simulink model "stepRecovery_compatibility"  (Simulink 8.3)
settings: Solver=ode3  SolverMode=SingleTasking  StartTime=0.0  StopTime="CONFIG.SIMULATION_TIME "  FixedStep=CONFIG.Ts  RelTol=1e-3
InitFcn:
  | cd(fileparts(which(bdroot)));
  | initStepRecovery;
values from neighbouring files (symbols this model uses):
  baseToWorldRotationPort = '/matlabTorqueBalancing/floatingBaseRotationMatrix:i'    [esperimento_fake2.mat]    (also in initStepRecovery.m = ['/' WBT_modelName '/floatingBaseRotationMatrix:i']; initTorqueBalancing.m = ['/' WBT_modelName '/floatingBaseRotationMatrix:i']; secondo_risultato.mat)
  bVectorConstraints = [0 0 0 0 0 0 0 0 0 0 0 0 ... (19 elements, 19x1)]    [esperimento_fake2.mat]    (also in secondo_risultato.mat)
  CONFIG =     [esperimento_fake2.mat]    (also in secondo_risultato.mat)
  ConstraintsMatrix = [3.73205080757 1 0.267949192431 -0.267949192431 -1 -3.73205080757 -3.73205080757 -1 -0.267949192431 0.267949192431 1 3.73205080757 ... (114 elements, 19x6)]    [esperimento_fake2.mat]    (also in secondo_risultato.mat)
  gain =     [esperimento_fake2.mat]    (also in secondo_risultato.mat)
  references =     [esperimento_fake2.mat]    (also in secondo_risultato.mat)
  reg =     [esperimento_fake2.mat]    (also in secondo_risultato.mat)
  ROBOT_DOF = 23    [esperimento_fake2.mat]    (also in secondo_risultato.mat)
  ROBOT_DOF_FOR_SIMULINK = [1 0 0 0 0 0 0 0 0 0 0 0 ... (529 elements, 23x23)]    [esperimento_fake2.mat]    (also in secondo_risultato.mat)
  sat =     [esperimento_fake2.mat]    (also in secondo_risultato.mat)
  SM =     [esperimento_fake2.mat]    (also in secondo_risultato.mat)
  sm =     [esperimento_fake2.mat]    (also in secondo_risultato.mat)
  WBT_modelName = 'matlabTorqueBalancing'    [esperimento_fake2.mat]    (also in initStepRecovery.m; initTorqueBalancing.m; secondo_risultato.mat)
  WBT_robotName = ''    [esperimento_fake2.mat]    (also in secondo_risultato.mat)
undefined symbols (not defined in the file or in its folder): bVectorConstraintsMPC, ConstraintsMatrixMPC, DiscIntNeverNeededParam, mpc_init
libraries: WBToolboxLibrary x191, simulink x22, simulink_extras x4
(part 6 of 6)

== system stepRecovery_compatibility/DesValues/State Machine Step Recovery/Step Recovery reference generator/Step Recovery Techniques /Capture Point Computer/Capture Point-alternative/omega ==
  COMx : Inport
  Constant : Constant  Value=9.81
  Divide : Product  Inputs=*/
  Selector : Selector  InputPortWidth=3  IndexOptions=Index vector (dialog)  Indices=[3]  OutputSizes=1
  Sqrt : Sqrt  SaturateOnIntegerOverflow=on
  holder 1 : WBToolboxLibrary/Utilities/holder 
  omega : Outport
  wires:
  Sqrt/1 -> omega/1
  Divide/1 -> Sqrt/1
  Constant/1 -> Divide/1
  holder 1/1 -> Divide/2
  Selector/1 -> holder 1/1
  COMx/1 -> Selector/1

== system stepRecovery_compatibility/DesValues/State Machine Step Recovery/Step Recovery reference generator/Step Recovery Techniques /Capture Point Computer/ICP /omega ==
  COMx : Inport
  Constant : Constant  Value=9.81
  Divide : Product  Inputs=*/
  Selector : Selector  InputPortWidth=3  IndexOptions=Index vector (dialog)  Indices=[3]  OutputSizes=1
  Sqrt : Sqrt  SaturateOnIntegerOverflow=on
  holder 1 : WBToolboxLibrary/Utilities/holder 
  omega : Outport
  wires:
  COMx/1 -> Selector/1
  Selector/1 -> holder 1/1
  holder 1/1 -> Divide/2
  Constant/1 -> Divide/1
  Divide/1 -> Sqrt/1
  Sqrt/1 -> omega/1

== system stepRecovery_compatibility/DesValues/State Machine Step Recovery/Step Recovery reference generator/Inverse Kinematics/Pseudo-Inverse kinematics Solver/From guess to q_ikin/l_sole_H_root_link1/Visualize hom transf4 ==
  H : Inport
  "CoM6D ->  CoMXYZ1" : Selector  NumberOfDimensions=2  InputPortWidth=7  IndexOptions=Index vector (dialog),Index vector (dialog)  Indices=[1 2 3],[1 2 3]  OutputSizes=1,1
  "CoM6D ->  CoMXYZ2" : Selector  NumberOfDimensions=2  InputPortWidth=7  IndexOptions=Index vector (dialog),Index vector (dialog)  Indices=[1 2 3],[4]  OutputSizes=1,1
  Hom : Scope
      settings: TimeRange=auto  ShowLegends=on  MaxDataPoints=5000  SaveToWorkspace=off  SaveName=ScopeData3  YMin=-1.25  YMax=1.25  SampleTime=-1
  R : Scope
      settings: TimeRange=auto  MaxDataPoints=5000  SaveToWorkspace=off  YMin=-0.125  YMax=1.125  SampleTime=-1
  p : Scope
      settings: TimeRange=auto  MaxDataPoints=5000  SaveToWorkspace=off  SaveName=ScopeData2  YMin=-1.00000  YMax=1.00000  SampleTime=-1
  wires:
  H/1 -> "CoM6D ->  CoMXYZ1"/1, Hom/1, "CoM6D ->  CoMXYZ2"/1
  "CoM6D ->  CoMXYZ2"/1 -> p/1
  "CoM6D ->  CoMXYZ1"/1 -> R/1

== system stepRecovery_compatibility/DesValues/State Machine Step Recovery/Step Recovery reference generator/Inverse Kinematics/Pseudo-Inverse kinematics Solver/From guess to q_ikin/l_sole_H_root_link2/Visualize hom transf4 ==
  H : Inport
  "CoM6D ->  CoMXYZ1" : Selector  NumberOfDimensions=2  InputPortWidth=7  IndexOptions=Index vector (dialog),Index vector (dialog)  Indices=[1 2 3],[1 2 3]  OutputSizes=1,1
  "CoM6D ->  CoMXYZ2" : Selector  NumberOfDimensions=2  InputPortWidth=7  IndexOptions=Index vector (dialog),Index vector (dialog)  Indices=[1 2 3],[4]  OutputSizes=1,1
  Hom : Scope
      settings: TimeRange=auto  ShowLegends=on  MaxDataPoints=5000  SaveToWorkspace=off  SaveName=ScopeData3  YMin=-1.25  YMax=1.25  SampleTime=-1
  R : Scope
      settings: TimeRange=auto  MaxDataPoints=5000  SaveToWorkspace=off  YMin=-0.125  YMax=1.125  SampleTime=-1
  p : Scope
      settings: TimeRange=auto  MaxDataPoints=5000  SaveToWorkspace=off  SaveName=ScopeData2  YMin=-1.00000  YMax=1.00000  SampleTime=-1
  wires:
  H/1 -> "CoM6D ->  CoMXYZ1"/1, Hom/1, "CoM6D ->  CoMXYZ2"/1
  "CoM6D ->  CoMXYZ2"/1 -> p/1
  "CoM6D ->  CoMXYZ1"/1 -> R/1

== matlab function DesValues/State Machine/visualise inertial/w_H_root_link1/fromImuToHomogeousTransformFCN ==
  data: imu_H_link input double; imu_H_link_0 input double; link_H_root input double; inertial_0 input double; inertial input double; neck input double; w_H_root output double; CONFIG parameter double
function w_H_root = fromBaseToWorldWithImuFCN(imu_H_link,imu_H_link_0,link_H_root,inertial_0,inertial,neck,CONFIG)
%#codegen
w_H_root = fromBaseToWorldWithImu(imu_H_link,imu_H_link_0,link_H_root,inertial_0,inertial,neck,CONFIG);

== matlab function DesValues/Internal coordinator/w_H_root_link4/fromImuToHomogeousTransformFCN ==
  data: imu_H_link input double; imu_H_link_0 input double; link_H_root input double; inertial_0 input double; inertial input double; neck input double; w_H_root output double; CONFIG parameter double
function w_H_root = fromBaseToWorldWithImuFCN(imu_H_link,imu_H_link_0,link_H_root,inertial_0,inertial,neck,CONFIG)
%#codegen
w_H_root = fromBaseToWorldWithImu(imu_H_link,imu_H_link_0,link_H_root,inertial_0,inertial,neck,CONFIG);

== matlab function DesValues/MATLAB Function ==
  data: w_H_b_vectorised input double; w_H_b output double; foot_p_b input double; rollPitchYaw output double
function [w_H_b,rollPitchYaw] = buildHomogenousTranformation(w_H_b_vectorised,foot_p_b)
%#codegen

w_H_b = [w_H_b_vectorised(1:4),w_H_b_vectorised(5:8),w_H_b_vectorised(9:12),...
         w_H_b_vectorised(13:16)];

w_H_b(1:3,4) = foot_p_b;
rollPitchYaw = rollPitchYawFromRotation(w_H_b(1:3,1:3));
rollPitchYaw(3) = 0;

== matlab function controller_QP/integralOf Hw/MATLAB Function ==
  data: qjErr input double; dqjEquivalent output double; Jc input double; vbEquivalent output double
function [dqjEquivalent, vbEquivalent] = generateReferencesForH(qjErr,Jc)
%#codegen

dqjEquivalent = qjErr;
vbEquivalent  = -eye(6)/Jc(1:6,1:6)*Jc(1:6,7:end)*qjErr;

end

== matlab function DesValues/State Machine Walking/nu/MATLAB Function ==
  data: JcLeftFoot input double; JcRightFoot input double; activeFeetConstraints input double; y output double; qD input double; reg parameter double
function y = fcn(JcLeftFoot,JcRightFoot,activeFeetConstraints,qD,reg)
%#codegen

Jc = [activeFeetConstraints(1)*JcLeftFoot;
      activeFeetConstraints(2)*JcRightFoot];

pinvJb = (Jc(:,1:6)'*Jc(:,1:6) + reg.pinvDampVb*eye(6))\Jc(:,1:6)';  
  
% pinvJb = pinv(Jc(:,1:6));

y = -pinvJb*Jc(:,7:end)*qD;

== matlab function DesValues/State Machine Walking/stateMachineFCN ==
  data: connection input double; wrench_rightFoot input double; wrench_leftFoot input double; CoM_0 input double; q0 input double; w_CoM input double; CoMIn input double; qIn input double; constraintsIn input double; w_H_b output double; CoMDes output double; qDes output double; constraints output double; l_sole_H_b input double; r_sole_H_b input double; sm parameter double; impedances output double; gain parameter double; currentState output double
function [w_H_b, CoMDes,qDes,constraints,impedances,currentState] = ...
    stateMachineFCN(connection,wrench_rightFoot,wrench_leftFoot,CoM_0, q0, w_CoM , CoMIn, qIn, constraintsIn, l_sole_H_b, r_sole_H_b, sm,gain)
%#codegen
 
[CoMDes,qDes,constraints, currentState,impedances,w_H_b] = ...
    stateMachineWalking(connection,CoM_0, q0, w_CoM, CoMIn, qIn, constraintsIn, wrench_rightFoot,wrench_leftFoot,l_sole_H_b, r_sole_H_b, sm,gain);

== matlab function DesValues/Internal coordinator/nu/MATLAB Function ==
  data: JcLeftFoot input double; JcRightFoot input double; activeFeetConstraints input double; y output double; qD input double; reg parameter double
function y = fcn(JcLeftFoot,JcRightFoot,activeFeetConstraints,qD,reg)
%#codegen

Jc = [activeFeetConstraints(1)*JcLeftFoot;
      activeFeetConstraints(2)*JcRightFoot];

pinvJb = (Jc(:,1:6)'*Jc(:,1:6) + reg.pinvDampVb*eye(6))\Jc(:,1:6)';  
  
% pinvJb = pinv(Jc(:,1:6));

y = -pinvJb*Jc(:,7:end)*qD;

== matlab function DesValues/State Machine/w_H_root_link4/fromImuToHomogeousTransformFCN ==
  data: imu_H_link input double; imu_H_link_0 input double; link_H_root input double; inertial_0 input double; inertial input double; neck input double; w_H_root output double; CONFIG parameter double
function w_H_root = fromBaseToWorldWithImuFCN(imu_H_link,imu_H_link_0,link_H_root,inertial_0,inertial,neck,CONFIG)
%#codegen
w_H_root = fromBaseToWorldWithImu(imu_H_link,imu_H_link_0,link_H_root,inertial_0,inertial,neck,CONFIG);

== matlab function DesValues/State Machine/w_H_root_link1/fromImuToHomogeousTransformFCN ==
  data: imu_H_link input double; imu_H_link_0 input double; link_H_root input double; inertial_0 input double; inertial input double; neck input double; w_H_root output double; CONFIG parameter double
function w_H_root = fromBaseToWorldWithImuFCN(imu_H_link,imu_H_link_0,link_H_root,inertial_0,inertial,neck,CONFIG)
%#codegen
w_H_root = fromBaseToWorldWithImu(imu_H_link,imu_H_link_0,link_H_root,inertial_0,inertial,neck,CONFIG);

== matlab function DesValues/Internal coordinator/refGen/refGenFCN ==
  data: xCom0 input double; qDes output double; q0 input double; t input double; references parameter double; desired_x_dx_ddx_CoM output double
function [qDes,desired_x_dx_ddx_CoM] = refGenFCN(xCom0,q0,t,references)
%#codegen

[qDes,desired_x_dx_ddx_CoM] = refGen(xCom0,q0,t,references);

== matlab function DesValues/State Machine Walking/w_H_root_link4/fromImuToHomogeousTransformFCN ==
  data: imu_H_link input double; imu_H_link_0 input double; link_H_root input double; inertial_0 input double; inertial input double; neck input double; w_H_root output double; CONFIG parameter double
function w_H_root = fromBaseToWorldWithImuFCN(imu_H_link,imu_H_link_0,link_H_root,inertial_0,inertial,neck,CONFIG)
%#codegen
w_H_root = fromBaseToWorldWithImu(imu_H_link,imu_H_link_0,link_H_root,inertial_0,inertial,neck,CONFIG);

== matlab function DesValues/State Machine/nu/MATLAB Function ==
  data: JcLeftFoot input double; JcRightFoot input double; activeFeetConstraints input double; y output double; qD input double; reg parameter double
function y = fcn(JcLeftFoot,JcRightFoot,activeFeetConstraints,qD,reg)
%#codegen

Jc = [activeFeetConstraints(1)*JcLeftFoot;
      activeFeetConstraints(2)*JcRightFoot];

pinvJb = pinvDamped(Jc(:,1:6),reg.pinvDampVb);  
  
% pinvJb = pinv(Jc(:,1:6));

y = -pinvJb*Jc(:,7:end)*qD;

== matlab function DesValues/State Machine/stateMachineFCN ==
  data: wrench_rightFoot input double; wrench_leftFoot input double; w_H_b output double; CoMDes output double; qDes output double; constraints output double; CoM_0 input double; q0 input double; l_sole_CoM input double; r_sole_CoM input double; qj input double; t input double; l_sole_H_b input double; r_sole_H_b input double; sm parameter double; impedances output double; kpCom output double; kdCom output double; gain parameter double; currentState output double; jointsSmoothingTime output double
function [w_H_b, CoMDes,qDes,constraints,impedances,kpCom,kdCom,currentState,jointsSmoothingTime] = ...
    stateMachineFCN(wrench_rightFoot,wrench_leftFoot,CoM_0, q0, l_sole_CoM,r_sole_CoM,qj, t, l_sole_H_b, r_sole_H_b, sm,gain)
%#codegen
 
[w_H_b, CoMDes,qDes,constraints,impedances,kpCom,kdCom,currentState,jointsSmoothingTime] = ...
    stateMachine(CoM_0, q0, l_sole_CoM,r_sole_CoM,qj, t, wrench_rightFoot,wrench_leftFoot,l_sole_H_b, r_sole_H_b, sm,gain);

== matlab function DesValues/State Machine Walking/w_H_root_link1/fromImuToHomogeousTransformFCN ==
  data: imu_H_link input double; imu_H_link_0 input double; link_H_root input double; inertial_0 input double; inertial input double; neck input double; w_H_root output double; CONFIG parameter double
function w_H_root = fromBaseToWorldWithImuFCN(imu_H_link,imu_H_link_0,link_H_root,inertial_0,inertial,neck,CONFIG)
%#codegen
w_H_root = fromBaseToWorldWithImu(imu_H_link,imu_H_link_0,link_H_root,inertial_0,inertial,neck,CONFIG);

== matlab function Dump and visualize/plotNorms/norm ==
  data: u input double; normU output double
function normU = fcn(u)
%#codegen

normU = norm(u);

== matlab function Dump and visualize/plotNorms/norm1 ==
  data: u input double; normU output double
function normU = fcn(u)
%#codegen

normU = norm(u);

== matlab function controller_QP/tau(f)  ==
  data: tauModel output double; Sigma output double; NA output double; fHdotDesC1C2 output double; HessianMatrixQP1Foot output double; gradientQP1Foot output double; ConstraintsMatrixQP1Foot output double; bVectorConstraintsQp1Foot output double; HessianMatrixQP2Feet output double; gradientQP2Feet output double; ConstraintsMatrixQP2Feet output double; bVectorConstraintsQp2Feet output double; constraints input double; ROBOT_DOF_FOR_SIMULINK input double; ConstraintsMatrix input double; bVectorConstraints input double; q input double; qDes input double; v input double; M input double; h input double; H input double; intHw input double; w_H_l_sole input double; w_H_r_sole input double; JL input double; JR input double; dJLv input double; dJRv input double; xcom input double; J_CoM input double; desired_x_dx_ddx_CoM input double; gainsPCOM input double; gainsDCOM input double; impedances input double; r_fin input double; r_init input double; r_icp input double; ENABLE_cop input double; intErrorCoM input double; ki_int_qtilde input double; reg parameter double; gain parameter double; errorCoM output double; qTilde output double; f output double
function [tauModel,Sigma,NA,fHdotDesC1C2, ...
          HessianMatrixQP1Foot,gradientQP1Foot,ConstraintsMatrixQP1Foot,bVectorConstraintsQp1Foot,...
          HessianMatrixQP2Feet,gradientQP2Feet,ConstraintsMatrixQP2Feet,bVectorConstraintsQp2Feet,...
          errorCoM,qTilde,f]    =  ...
          balancingControllerFCN(constraints,ROBOT_DOF_FOR_SIMULINK,ConstraintsMatrix,bVectorConstraints,...
          q,qDes,v, M, h , H,intHw,w_H_l_sole, w_H_r_sole, JL,JR, dJLv,dJRv, xcom,J_CoM, desired_x_dx_ddx_CoM,...
          gainsPCOM,gainsDCOM,impedances,r_fin,r_init,r_icp,ENABLE_cop, intErrorCoM,ki_int_qtilde,reg,gain)
%#codegen
    [tauModel,Sigma,NA,fHdotDesC1C2, ...
                  HessianMatrixQP1Foot,gradientQP1Foot,ConstraintsMatrixQP1Foot,bVectorConstraintsQp1Foot,...
                  HessianMatrixQP2Feet,gradientQP2Feet,ConstraintsMatrixQP2Feet,bVectorConstraintsQp2Feet,...
                  errorCoM,qTilde,f]    =  ...
                  balancingControllerStep(constraints,ROBOT_DOF_FOR_SIMULINK,ConstraintsMatrix,bVectorConstraints,...
                        q,qDes,v, M, h , H,intHw,w_H_l_sole, w_H_r_sole, JL,JR, dJLv,dJRv, xcom,J_CoM, desired_x_dx_ddx_CoM,...
                        gainsPCOM,gainsDCOM,impedances,r_fin,r_init,r_icp,ENABLE_cop,intErrorCoM,ki_int_qtilde,reg,gain);
end

== matlab function emergency stop: joint limits/MATLAB Function ==
  data: umin input double; umax input double; u input double; inRange output double; tol input double
function inRange = checkRange(umin, umax, u, tol)
%#codegen

res = u < umin + tol | u > umax - tol;
res = sum(res);
if res==0
    inRange = 1;
else
    inRange = 0;
    u < umin + tol | u > umax - tol
end

== matlab function DesValues/State Machine Step Recovery/nu/MATLAB Function ==
  data: JcLeftFoot input double; JcRightFoot input double; activeFeetConstraints input double; y output double; qD input double; reg parameter double
function y = fcn(JcLeftFoot,JcRightFoot,activeFeetConstraints,qD,reg)
%#codegen

Jc = [activeFeetConstraints(1)*JcLeftFoot;
      activeFeetConstraints(2)*JcRightFoot];

pinvJb = pinvDamped(Jc(:,1:6),reg.pinvDampVb);  
  
% pinvJb = pinv(Jc(:,1:6));

y = -pinvJb*Jc(:,7:end)*qD;

== matlab function controller_QP/integralOf Hw/MATLAB Function1 ==
  data: H input double; deltaPhi output double
function deltaPhi = generateCentroidalOrient(H)
%#codegen

deltaPhi = H(4:end);

end

== matlab function DesValues/State Machine/visualise inertial/Visualize hom transf1/MATLAB Function ==
  data: R input double; rollPitchYaw output double
function rollPitchYaw = buildHomogenousTranformation(R)
%#codegen

rollPitchYaw = rollPitchYawFromRotation(R);

rollPitchYaw = rollPitchYaw*180/pi;

== matlab function DesValues/State Machine/visualise inertial/Visualize hom transf2/MATLAB Function ==
  data: R input double; rollPitchYaw output double
function rollPitchYaw = buildHomogenousTranformation(R)
%#codegen

rollPitchYaw = rollPitchYawFromRotation(R);

rollPitchYaw = rollPitchYaw*180/pi;

== matlab function DesValues/State Machine/visualise inertial/Visualize hom transf4/MATLAB Function ==
  data: R input double; rollPitchYaw output double
function rollPitchYaw = buildHomogenousTranformation(R)
%#codegen

rollPitchYaw = rollPitchYawFromRotation(R);

rollPitchYaw = rollPitchYaw*180/pi;

== matlab function DesValues/State Machine/visualise inertial/Visualize hom transf5/MATLAB Function ==
  data: R input double; rollPitchYaw output double
function rollPitchYaw = buildHomogenousTranformation(R)
%#codegen

rollPitchYaw = rollPitchYawFromRotation(R);

rollPitchYaw = rollPitchYaw*180/pi;

== matlab function DesValues/State Machine/visualise inertial/Visualize hom transf6/MATLAB Function ==
  data: R input double; rollPitchYaw output double
function rollPitchYaw = buildHomogenousTranformation(R)
%#codegen

rollPitchYaw = rollPitchYawFromRotation(R);

rollPitchYaw = rollPitchYaw*180/pi;

== matlab function DesValues/State Machine/visualise inertial/Visualize hom transf3/MATLAB Function ==
  data: R input double; rollPitchYaw output double
function rollPitchYaw = buildHomogenousTranformation(R)
%#codegen

rollPitchYaw = rollPitchYawFromRotation(R);

rollPitchYaw = rollPitchYaw*180/pi;

== matlab function DesValues/State Machine/visualise inertial/w_H_root_link4/fromImuToHomogeousTransformFCN ==
  data: imu_H_link input double; imu_H_link_0 input double; link_H_root input double; inertial_0 input double; inertial input double; neck input double; w_H_root output double; CONFIG parameter double
function w_H_root = fromBaseToWorldWithImuFCN(imu_H_link,imu_H_link_0,link_H_root,inertial_0,inertial,neck,CONFIG)
%#codegen
w_H_root = fromBaseToWorldWithImu(imu_H_link,imu_H_link_0,link_H_root,inertial_0,inertial,neck,CONFIG);

== matlab function DesValues/State Machine Step Recovery/stateMachineFCN ==
  data: wrench_rightFoot input double; wrench_leftFoot input double; w_H_b output double; CoMDes output double; qDes output double; constraints output double; CoM_0 input double; q0 input double; l_sole_CoM input double; r_sole_CoM input double; qj input double; t input double; l_sole_H_b input double; r_sole_H_b input double; sm parameter double; impedances output double; kpCom output double; kdCom output double; gain parameter double; currentState output double; jointsSmoothingTime output double; STEP_DOWN input double; COM_l_v input double; r_CxP input double; MAKE_A_STEP input double; QP_OFF output double; SMOOTH output double; SMOOTH_com output double; q_step input double; COM_ref input double; l_solex input double; r_solex input double
function [w_H_b, CoMDes,qDes,constraints,impedances,kpCom,kdCom,currentState,jointsSmoothingTime, QP_OFF, SMOOTH, SMOOTH_com] = ...
    stateMachineFCN(wrench_rightFoot,wrench_leftFoot,CoM_0, q0, l_sole_CoM,r_sole_CoM,qj, t, l_sole_H_b, r_sole_H_b, sm,gain, STEP_DOWN, COM_l_v, r_CxP, MAKE_A_STEP, q_step, COM_ref, l_solex, r_solex)
%#codegen
 
[w_H_b, CoMDes,qDes,constraints,impedances,kpCom,kdCom,currentState,jointsSmoothingTime, QP_OFF, SMOOTH, SMOOTH_com] = ...
    stateMachineStep(CoM_0, q0, l_sole_CoM,r_sole_CoM,qj, t, wrench_rightFoot,wrench_leftFoot,l_sole_H_b, r_sole_H_b, sm,gain, STEP_DOWN, r_CxP, COM_l_v, MAKE_A_STEP, q_step, COM_ref, l_solex, r_solex);

== matlab function DesValues/State Machine Step Recovery/visualise inertial/Visualize hom transf1/MATLAB Function ==
  data: R input double; rollPitchYaw output double
function rollPitchYaw = buildHomogenousTranformation(R)
%#codegen

rollPitchYaw = rollPitchYawFromRotation(R);

rollPitchYaw = rollPitchYaw*180/pi;

== matlab function DesValues/State Machine Step Recovery/visualise inertial/Visualize hom transf2/MATLAB Function ==
  data: R input double; rollPitchYaw output double
function rollPitchYaw = buildHomogenousTranformation(R)
%#codegen

rollPitchYaw = rollPitchYawFromRotation(R);

rollPitchYaw = rollPitchYaw*180/pi;

== matlab function DesValues/State Machine Step Recovery/visualise inertial/Visualize hom transf3/MATLAB Function ==
  data: R input double; rollPitchYaw output double
function rollPitchYaw = buildHomogenousTranformation(R)
%#codegen

rollPitchYaw = rollPitchYawFromRotation(R);

rollPitchYaw = rollPitchYaw*180/pi;

== matlab function DesValues/State Machine Step Recovery/visualise inertial/Visualize hom transf4/MATLAB Function ==
  data: R input double; rollPitchYaw output double
function rollPitchYaw = buildHomogenousTranformation(R)
%#codegen

rollPitchYaw = rollPitchYawFromRotation(R);

rollPitchYaw = rollPitchYaw*180/pi;

== matlab function DesValues/State Machine Step Recovery/visualise inertial/Visualize hom transf5/MATLAB Function ==
  data: R input double; rollPitchYaw output double
function rollPitchYaw = buildHomogenousTranformation(R)
%#codegen

rollPitchYaw = rollPitchYawFromRotation(R);

rollPitchYaw = rollPitchYaw*180/pi;

== matlab function DesValues/State Machine Step Recovery/visualise inertial/Visualize hom transf6/MATLAB Function ==
  data: R input double; rollPitchYaw output double
function rollPitchYaw = buildHomogenousTranformation(R)
%#codegen

rollPitchYaw = rollPitchYawFromRotation(R);

rollPitchYaw = rollPitchYaw*180/pi;

== matlab function DesValues/State Machine Step Recovery/visualise inertial/w_H_root_link1/fromImuToHomogeousTransformFCN ==
  data: imu_H_link input double; imu_H_link_0 input double; link_H_root input double; inertial_0 input double; inertial input double; neck input double; w_H_root output double; CONFIG parameter double
function w_H_root = fromBaseToWorldWithImuFCN(imu_H_link,imu_H_link_0,link_H_root,inertial_0,inertial,neck,CONFIG)
%#codegen
w_H_root = fromBaseToWorldWithImu(imu_H_link,imu_H_link_0,link_H_root,inertial_0,inertial,neck,CONFIG);

== matlab function DesValues/State Machine Step Recovery/visualise inertial/w_H_root_link4/fromImuToHomogeousTransformFCN ==
  data: imu_H_link input double; imu_H_link_0 input double; link_H_root input double; inertial_0 input double; inertial input double; neck input double; w_H_root output double; CONFIG parameter double
function w_H_root = fromBaseToWorldWithImuFCN(imu_H_link,imu_H_link_0,link_H_root,inertial_0,inertial,neck,CONFIG)
%#codegen
w_H_root = fromBaseToWorldWithImu(imu_H_link,imu_H_link_0,link_H_root,inertial_0,inertial,neck,CONFIG);

== matlab function DesValues/State Machine Step Recovery/w_H_root_link1/fromImuToHomogeousTransformFCN ==
  data: imu_H_link input double; imu_H_link_0 input double; link_H_root input double; inertial_0 input double; inertial input double; neck input double; w_H_root output double; CONFIG parameter double
function w_H_root = fromBaseToWorldWithImuFCN(imu_H_link,imu_H_link_0,link_H_root,inertial_0,inertial,neck,CONFIG)
%#codegen
w_H_root = fromBaseToWorldWithImu(imu_H_link,imu_H_link_0,link_H_root,inertial_0,inertial,neck,CONFIG);

== matlab function DesValues/State Machine Step Recovery/w_H_root_link4/fromImuToHomogeousTransformFCN ==
  data: imu_H_link input double; imu_H_link_0 input double; link_H_root input double; inertial_0 input double; inertial input double; neck input double; w_H_root output double; CONFIG parameter double
function w_H_root = fromBaseToWorldWithImuFCN(imu_H_link,imu_H_link_0,link_H_root,inertial_0,inertial,neck,CONFIG)
%#codegen
w_H_root = fromBaseToWorldWithImu(imu_H_link,imu_H_link_0,link_H_root,inertial_0,inertial,neck,CONFIG);

== matlab function DesValues/State Machine Step Recovery/Step Recovery reference generator/Step Recovery Techniques /FPE module/MATLAB Function ==
  data: base_origin input double; Mbb input double; Mbb_COM output double; COMx input double
function Mbb_COM  = COM_inertia_matrix_sim(base_origin, Mbb, COMx)
Mbb_COM = COM_inertia_matrix(Mbb, base_origin, COMx);

== matlab function DesValues/State Machine Step Recovery/Step Recovery reference generator/Step Recovery Techniques /Capture Point Computer/Capture Point-alternative/MATLAB Function ==
  data: omega input double; r_CP output double; r_ic input double; r_CxP input double; robot_step_time input double; STEP input double; delta_t input double
function r_CP = capture_point(omega, r_ic, r_CxP, robot_step_time, STEP, delta_t)
 persistent elapsed_time;
 
 if isempty(elapsed_time)
     elapsed_time = 0;
 end
 
 if (STEP == 0)
     r_CP = r_ic;
     elapsed_time = 0;
 
 else  r_CP = (r_ic - r_CxP)*exp(omega * (robot_step_time-elapsed_time)) + r_CxP;
       if (elapsed_time < (robot_step_time-delta_t))
           elapsed_time = elapsed_time + delta_t;
       end
 end
end

== matlab function DesValues/State Machine Step Recovery/Step Recovery reference generator/Step Recovery Techniques /Capture Point Computer/Capture Point-Pratt /MATLAB Function ==
  data: omega input double; r_CP output double; r_ic input double; robot_step_time input double; STEP input double; w_H_f input double; foot_size input double; T1 output double; T2 output double
function [r_CP, T1,T2] = capture_point(omega, r_ic, robot_step_time, STEP, w_H_f, foot_size)

 persistent r_ic0;
 
 if isempty(r_ic0)
     r_ic0 = r_ic;
 end

xm = foot_size(1,1);
xM = foot_size(1,2);
ym = foot_size(2,1);
yM = foot_size(2,2);

P1 = [xM;yM;0];
P2 = [xM;ym;0];
P3 = [xm;ym;0];
P4 = [xm;yM;0];

R = w_H_f(1:3,1:3);
p = w_H_f(1:3,4);

f_H_w = [R',        -R'*p;
        zeros(1,3),     1];
    
r_ic_local = f_H_w*[r_ic;1];


if (STEP == 0)
    r_CP = r_ic;
    r_ic0 = r_ic;
    T1 = zeros(3,1);
    T2 = zeros(3,1);
    
else if (r_ic_local(2) < 0)
        T1 = (r_ic0 - P2)*exp(omega * robot_step_time) + P2;
        T2 = (r_ic0 - P3)*exp(omega * robot_step_time) + P3;
        r_CP_temp = w_H_f*[max(T1(1),T2(1)) - xM; min(T1(2),T2(2))+ym;0;1];
        r_CP = r_CP_temp(1:3);       
        
    else
        T1 = (r_ic0 - P1)*exp(omega * robot_step_time) + P1;
        T2 = (r_ic0 - P4)*exp(omega * robot_step_time) + P4;
        r_CP_temp = w_H_f*[max(T1(1),T2(1)) - xM; max(T1(2),T2(2))+yM;0;1];
        r_CP = r_CP_temp(1:3); 
    end
end
end

== matlab function DesValues/State Machine Step Recovery/Step Recovery reference generator/Step Recovery Techniques /FPE module/MATLAB Function2 ==
  data: COM_vel input double; m input double; J_COM input double; COMx input double; g input double; theta_bar output double; foot input double; x output double; fpe_poly output double; fpe_poly_offset output double; dissipation output double; offset input double
function [theta_bar, x, fpe_poly, fpe_poly_offset, dissipation] = fpe_sim(COM_vel, m, J_COM, COMx, g, foot, offset)
 [theta_bar, x, fpe_poly, fpe_poly_offset, dissipation] = fpe_computation(m, COMx, COM_vel, J_COM, g, foot, offset);
end

== matlab function DesValues/State Machine Step Recovery/Step Recovery reference generator/Step Recovery Techniques /FPE module/Out of left foot_CH/Inverse ==
  data: w_H_a input double; a_H_w output double
function a_H_w = inverse(w_H_a)

R = w_H_a(1:3,1:3);
p = w_H_a(1:3,4);

a_H_w = [R',        -R'*p;
        zeros(1,3),     1];

== matlab function DesValues/State Machine Step Recovery/Step Recovery reference generator/Step Recovery Techniques /Capture Point Computer/Out of left foot_CH/Inverse ==
  data: w_H_a input double; a_H_w output double
function a_H_w = inverse(w_H_a)

R = w_H_a(1:3,1:3);
p = w_H_a(1:3,4);

a_H_w = [R',        -R'*p;
        zeros(1,3),     1];

== matlab function DesValues/State Machine Step Recovery/Step Recovery reference generator/Step Recovery Techniques /FPE module/Out of left foot_CH/MATLAB Function ==
  data: x input double; OUT output double; w_H_lsole input double; w_H_rsole input double; foot_size input double
function OUT = in_convex_hull(x,w_H_lsole, w_H_rsole, foot_size)
OUT = in_convex_hull(x,w_H_lsole, w_H_rsole, foot_size);

== matlab function DesValues/State Machine Step Recovery/Step Recovery reference generator/Step Recovery Techniques /Capture Point Computer/Capture Point/MATLAB Function1 ==
  data: omega input double; r input double; r_eq output double; delta_t input double; OUT input double
function r_eq = equivalent_r (omega, r, delta_t, OUT)
r_eq = equivalent_r (r, delta_t, omega, OUT);

== matlab function DesValues/State Machine Step Recovery/Step Recovery reference generator/Step Recovery Techniques /Capture Point Computer/Capture Point/MATLAB Function ==
  data: omega input double; r_CP output double; r_ic input double; r_CxP input double; robot_step_time input double; STEP input double; r_ic0 output double
function [r_CP, r_ic0] = capture_point(omega, r_ic, r_CxP, robot_step_time, STEP)
[r_CP, r_ic0] = capture_point(STEP, r_ic, r_CxP, omega, robot_step_time);

== matlab function DesValues/State Machine Step Recovery/Step Recovery reference generator/Inverse Kinematics/MATLAB Function ==
  data: des_pos input double; w_H_f output double; rot_x input double; rot_y input double; rot_z input double
function w_H_f = desired_transformation (des_pos,rot_x, rot_y, rot_z)

des_pos = reshape(des_pos,3,1);
R=eul2rotm([rot_z,rot_y,rot_x]);

w_H_f = [R    ,des_pos; 
         zeros(1,3),1];

== matlab function DesValues/State Machine Step Recovery/Step Recovery reference generator/Step Recovery Techniques /ankle, CoP, Cmp (LEFT FOOT)/CMP computer/MATLAB Function ==
  data: R input double; s_A_b output double; p input double
function s_A_b = adjoint (R,p)
s_A_b = adjoint (R,p);

== matlab function DesValues/State Machine Step Recovery/Step Recovery reference generator/Step Recovery Techniques /Capture Point Computer/Capture Point/Versor ==
  data: r_CxP input double; omega input double; r_ic input double; r_ic_dot output double
function r_ic_dot = CP_direction(r_CxP, omega, r_ic)

r_ic_dot = omega*(r_ic - r_CxP);


end

== matlab function DesValues/State Machine Step Recovery/Step Recovery reference generator/Step Recovery Techniques /FPE module/Out of left foot_CH/Out of left foot  ==
  data: x input double; OUT output double; support input double; shadow input double; OUT_real output double
function [OUT, OUT_real] = exit_support_square_shadowed(x, support,shadow)
%computes whether x is outside the support polygon defined in supportp. x
%should be a two dimensional vector, while supportp a 2x2 matrix, where
%the first coloumn is the lower edge, while the first row corresponds to
%the first dimension of x. Notice that this check is done only if x is
%inside the shadowed region.
[OUT, OUT_real] = exit_support_square_shadowed(x, support, shadow);

== matlab function DesValues/State Machine Step Recovery/Step Recovery reference generator/Selector and Saturation/MATLAB Function ==
  data: x input double; x_sat output double; max_d input double; SAT output double; min_d input double
function [x_sat, SAT]=step_saturation(x,max_d,min_d)
[x_sat, SAT]=step_saturation(x,max_d,min_d);

== matlab function DesValues/State Machine Step Recovery/Step Recovery reference generator/Step Recovery Techniques /Capture Point Computer/Out of left foot_CH/MATLAB Function ==
  data: x input double; OUT output double; w_H_lsole input double; w_H_rsole input double; foot_size input double
function OUT = in_convex_hull(x,w_H_lsole, w_H_rsole, foot_size)
OUT = in_convex_hull(x,w_H_lsole, w_H_rsole, foot_size);

== matlab function DesValues/State Machine Step Recovery/Step Recovery reference generator/Step Recovery Techniques /Dump and Visualize SRT /MATLAB Function ==
  data: r_fin input double; COPx_tilde output double; r_init input double; r_icp input double
function COPx_tilde = projector(r_fin,r_init,r_icp)
L = sqrt((r_fin(1)-r_init(1))^2 + (r_fin(2)-r_init(2))^2);
    ctheta = 0;
    stheta = 0;
    if L > 0
        ctheta = (r_init(2)-r_fin(2))/L;
        stheta = (r_fin(1)-r_init(1))/L;
    end
COPx_tilde = ctheta*r_icp(1)+stheta*r_icp(2) -ctheta*r_init(1) - stheta*r_init(2);

== matlab function controller_QP/MATLAB Function ==
  data: r_fin input double; icpx_tilde output double; r_init input double; r_icp input double; f_qpg input double; cop_gain input double; cop_out output double; cop_ref output double; w_h_l input double
function [icpx_tilde, cop_out, cop_ref] = projector(r_fin,r_init,r_icp,f_qpg,cop_gain,w_h_l)
L = sqrt((r_fin(1)-r_init(1))^2 + (r_fin(2)-r_init(2))^2);
    ctheta = 0;
    stheta = 0;
    if L > 0
        ctheta = (r_init(2)-r_fin(2))/L;
        stheta = (r_fin(1)-r_init(1))/L;
    end
icpx_tilde = ctheta*r_icp(1)+stheta*r_icp(2) -ctheta*r_init(1) - stheta*r_init(2);
f_qp = zeros(6,1);
f_qp(1:3) = w_h_l(1:3,1:3)\f_qpg(1:3);
f_qp(4:6) = w_h_l(1:3,1:3)\f_qpg(4:6);

x_cop = -f_qp(5)/f_qp(3);
y_cop =  f_qp(4)/f_qp(3);

cop_out = ctheta*x_cop + stheta*y_cop;
cop_ref = (cop_gain +1)*(ctheta*r_icp(1)+stheta*r_icp(2)) + cop_gain*(-ctheta*r_init(1) - stheta*r_init(2));

== matlab function DesValues/State Machine Step Recovery/Step Recovery reference generator/Step Recovery Techniques /Capture Point Computer/Out of left foot_CH/Out of left foot  ==
  data: x input double; OUT output double; support input double; shadow input double; OUT_real output double
function [OUT, OUT_real] = exit_support_square_shadowed(x, support,shadow)
%computes whether x is outside the support polygon defined in supportp. x
%should be a two dimensional vector, while supportp a 2x2 matrix, where
%the first coloumn is the lower edge, while the first row corresponds to
%the first dimension of x. Notice that this check is done only if x is
%inside the shadowed region.
[OUT, OUT_real] = exit_support_square_shadowed(x, support, shadow);

== matlab function DesValues/State Machine Step Recovery/Step Recovery reference generator/Inverse Kinematics/Inverse ==
  data: w_H_a input double; a_H_w output double
function a_H_w = inverse(w_H_a)

R = w_H_a(1:3,1:3);
p = w_H_a(1:3,4);

a_H_w = [R',        -R'*p;
        zeros(1,3),     1];

== matlab function DesValues/State Machine Step Recovery/Visualize hom transf5/MATLAB Function ==
  data: R input double; rollPitchYaw output double
function rollPitchYaw = buildHomogenousTranformation(R)
%#codegen

rollPitchYaw = rollPitchYawFromRotation(R);

rollPitchYaw = rollPitchYaw*180/pi;

== matlab function controller_QP/MPC /MATLAB Function ==
  data: ConstraintsMatrix input double; bVectorConstraints input double; foot_size input double; dT input double; STEP input double; constraints_vec input double; w_H_l_sole input double; l_sole_H_r_sole input double; w_H_r_sole_in input double; COMx input double; COMv input double; Hw input double; COMdes input double; minZ input double; omega input double; f_prev input double; m input double; mpc_init parameter double; f output double; exitflag output double; COM_des output double; COMref output double
function [f,exitflag,COM_des,COMref] = mpc_step(ConstraintsMatrix, bVectorConstraints, foot_size, dT, STEP, constraints_vec, w_H_l_sole,l_sole_H_r_sole, w_H_r_sole_in, COMx, COMv, Hw, COMdes, minZ, omega, f_prev, m, mpc_init)
[f,exitflag,COM_des,COMref] = mpc_step(mpc_init,constraints_vec, ConstraintsMatrix, bVectorConstraints, w_H_l_sole,l_sole_H_r_sole, w_H_r_sole_in, COMx, COMv, Hw, COMdes, minZ, f_prev, foot_size, omega, m, dT, STEP);

== matlab function DesValues/State Machine Step Recovery/Step Recovery reference generator/Inverse Kinematics/Fill with zero ==
  data: u input double; y output double
function y = fill_zero(u)
y = zeros(length(u),3);
y(:,1) = u;

== matlab function DesValues/State Machine Step Recovery/Step Recovery reference generator/Inverse Kinematics/Pseudo-Inverse kinematics Solver/From guess to q_ikin/MATLAB Function1 ==
  data: s input double; s0 output double; reset input double
function s0 = holder(s, reset)
persistent state
%#codegen

if (isempty(state) || reset)
    state = s;
end

s0 = state;

== matlab function DesValues/State Machine Step Recovery/Step Recovery reference generator/Inverse Kinematics/Pseudo-Inverse kinematics Solver/q+base/MATLAB Function1 ==
  data: s input double; s0 output double; reset input double
function s0 = holder(s, reset)
persistent state
%#codegen

if (isempty(state) || reset)
    state = s;
end

s0 = state;

== matlab function DesValues/State Machine Step Recovery/Step Recovery reference generator/Inverse Kinematics/Fill with zero1 ==
  data: u input double; y output double
function y = fill_zero(u)
y = zeros(length(u),3);
y(:,1) = u;

== matlab function DesValues/State Machine Step Recovery/Step Recovery reference generator/Inverse Kinematics/MATLAB Function1 ==
  data: s input double; s0 output double; reset input double
function s0 = holder(s, reset)
persistent state
%#codegen

if (isempty(state) || reset)
    state = s;
end

s0 = state;

== matlab function DesValues/State Machine Step Recovery/Step Recovery reference generator/Inverse Kinematics/Pseudo-Inverse kinematics Solver/Generate ikin Errors/trajectoryGeneratorCoM ==
  data: lFootPos input double; rFootPos input double; rFootOri input double; lFootOri input double; cartesian_error input double; xCoM input double; qj input double; CoMRefsDes input double; posturesDes input double; lFootVel input double; rFootVel input double; dxCoM input double; dqj input double; iKinFeetCorr output double; iKinComCorr output double; iKinSoleCorr output double; iKinPostCorr output double; gain parameter double
function [iKinFeetCorr,iKinComCorr,iKinSoleCorr,iKinPostCorr]  = ikin_PosAndOriErrors(lFootPos,rFootPos,rFootOri,lFootOri,cartesian_error, xCoM, qj, CoMRefsDes,posturesDes,lFootVel,...
                                                                         rFootVel,dxCoM,dqj,gain)

[iKinFeetCorr,iKinComCorr,iKinSoleCorr,iKinPostCorr]  = ikin_PosAndOrientErrors(lFootPos,rFootPos,rFootOri,lFootOri,cartesian_error, xCoM,qj, CoMRefsDes,posturesDes,...
                                                                            lFootVel,rFootVel,dxCoM,dqj,gain);

end

== matlab function DesValues/State Machine Step Recovery/Step Recovery reference generator/Inverse Kinematics/Pseudo-Inverse kinematics Solver/ikin_DoubleIntegrator/BaseDerivative ==
  data: NuBase_Ref input double; BaseDer output double; baseQuat input double
function BaseDer   = BaseDeriv(NuBase_Ref, baseQuat)

BaseDer   = BaseDerivative(NuBase_Ref, baseQuat);

end

== matlab function DesValues/State Machine Step Recovery/Step Recovery reference generator/Inverse Kinematics/Pseudo-Inverse kinematics Solver/ikin_DoubleIntegrator/Define the base pose as pos+quat ==
  data: qRef_ikin_init input double; qRef_ikin_0 output double
function qRef_ikin_0 = ConvStateToQuat(qRef_ikin_init)

qRef_ikin_0 = convertStateToQuat(qRef_ikin_init);

end

== matlab function DesValues/State Machine Step Recovery/Step Recovery reference generator/Inverse Kinematics/Pseudo-Inverse kinematics Solver/ikin_DoubleIntegrator/Define the base pose as transformation matrix ==
  data: qRef_ikin_no_converted input double; qRef_ikin output double
function qRef_ikin = baseToTransMatr(qRef_ikin_no_converted)

qRef_ikin = BasePoseToTransMatrix(qRef_ikin_no_converted);

end

== matlab function DesValues/State Machine Step Recovery/Step Recovery reference generator/Inverse Kinematics/Pseudo-Inverse kinematics Solver/ikin_DoubleIntegrator/Joints references ==
  data: dNuRef_ikin input double; inverseKinRef output double; NuRef_ikin input double; qRef_ikin input double
function inverseKinRef = fcn(dNuRef_ikin, NuRef_ikin, qRef_ikin)

inverseKinRef = generateJointRef(dNuRef_ikin, NuRef_ikin, qRef_ikin);

end

== matlab function DesValues/State Machine Step Recovery/Step Recovery reference generator/Inverse Kinematics/Pseudo-Inverse kinematics Solver/ikin_utilities/ikin_forwardKin/FromFwdKin_ToPosAndOrient ==
  data: fwdkin_lfoot input double; fwdkin_rfoot input double; fwdkinCoM input double; fwdkin_rfootIni input double; delta_lfootPos output double; fwdkin_lfootIni input double; delta_lfootOri output double; delta_rfootPos output double; delta_rfootOri output double; CoMPos output double; lsole_H_rsole input double; rsole_H_lsole input double; cartesian_err output double
function [delta_lfootPos,delta_lfootOri,delta_rfootPos,delta_rfootOri,CoMPos,cartesian_err] = fromFdwKinToPosOri(fwdkin_lfoot,fwdkin_rfoot,fwdkinCoM,fwdkin_rfootIni,...
                                                                                                   fwdkin_lfootIni,lsole_H_rsole,rsole_H_lsole)

[delta_lfootPos,delta_lfootOri,delta_rfootPos,delta_rfootOri,CoMPos,cartesian_err] = fromFwdKinToPosAndOri(fwdkinCoM,fwdkin_lfoot,fwdkin_lfootIni,...
                                                                                             fwdkin_rfoot,fwdkin_rfootIni,lsole_H_rsole,rsole_H_lsole);
                                                                                         
end

== matlab function DesValues/State Machine Step Recovery/Step Recovery reference generator/Inverse Kinematics/Pseudo-Inverse kinematics Solver/trajectoryGeneratorCoM ==
  data: iKinFeetCorr input double; iKinComCorr input double; iKinSoleCorr input double; iKinPostCorr input double; J_lfoot input double; J_rfoot input double; J_com input double; dNuRef_ikin output double; dJcNu_lf input double; dJcNu_rf input double; dJ_comNu input double; constraints input double
function dNuRef_ikin   = ikin_AccelerationRef_generator(iKinFeetCorr, iKinComCorr, iKinSoleCorr, iKinPostCorr, J_lfoot, J_rfoot, J_com, dJcNu_lf,...
                                                       dJcNu_rf, dJ_comNu, constraints)

n_joints = size(J_com(:,7:end),2);

%% jacobians and jacobian derivatives
JFeet      = [constraints(1)*J_lfoot ; constraints(2)*J_rfoot];
JCoM       = J_com(1:3,:);
JPosture   = [zeros(n_joints,6),eye(n_joints)]; 

dJFeetNu   = [constraints(1)*dJcNu_lf; constraints(2)*dJcNu_rf];
dJCoMNu    = dJ_comNu(1:3);

Jsole      = [(1-constraints(1))*J_lfoot  ; (1-constraints(2))*J_rfoot];
dJsoleNu   = [(1-constraints(1))*dJcNu_lf ; (1-constraints(2))*dJcNu_rf];

%% state acceleration reference calculation
dNuRef_ikin = Ikin_AccelerationRef_generator(JFeet, JCoM, Jsole, JPosture, dJFeetNu, dJCoMNu, dJsoleNu, iKinFeetCorr, iKinComCorr, iKinSoleCorr, iKinPostCorr); 

end
